simulink model "Scenario_3_PF"  (R2020b)
settings: Solver=ode1  StartTime=0.0  StopTime=10.0  RelTol=1e-3
InitFcn:
  | Scenario_3_parameters;
values from neighbouring files (symbols this model uses):
  c0 = c0_zeb    (= 6.57988e-09)    [Scenario_17_parameters_v2.m]    (also in Scenario_1_parameters_v2.m; Scenario_2_parameters_v2.m; Scenario_3_parameters_v2.m)
  c0_hawk = 6.37282e-09    [Scenario_17_parameters_v2.m]    (also in Scenario_1_parameters_v2.m; Scenario_2_parameters_v2.m; Scenario_3_parameters_v2.m)
  c1 = c1_zeb    (= 9.15905e-09)    [Scenario_17_parameters_v2.m]    (also in Scenario_1_parameters_v2.m; Scenario_2_parameters_v2.m; Scenario_3_parameters_v2.m)
  c1_hawk = 8.76156e-09    [Scenario_17_parameters_v2.m]    (also in Scenario_1_parameters_v2.m; Scenario_2_parameters_v2.m; Scenario_3_parameters_v2.m)
  fg = 50    [Scenario_17_parameters_v2.m]    (also in Scenario_1_parameters_v2.m; Scenario_2_parameters_v2.m; Scenario_3_parameters_v2.m)
  G10gen = 0.90    (= 0.9)    [Scenario_3_parameters_v2.m]
  G12gen = 0.85    [Scenario_3_parameters_v2.m]
  G1gen = 0.4692    [Scenario_17_parameters_v2.m]    (also in Scenario_1_parameters_v2.m = 0.1; Scenario_2_parameters_v2.m = 0.298581; Scenario_3_parameters_v2.m = 0.65)
  G2gen = 0.80    (= 0.8)    [Scenario_1_parameters_v2.m]    (also in Scenario_2_parameters_v2.m = 0.7; Scenario_3_parameters_v2.m = 0.4)
  G3gen = 0.85    [Scenario_1_parameters_v2.m]    (also in Scenario_2_parameters_v2.m = 0.9; Scenario_3_parameters_v2.m = 0.6)
  G4gen = 0.65    [Scenario_3_parameters_v2.m]
  G5gen = 0.75    [Scenario_17_parameters_v2.m]    (also in Scenario_1_parameters_v2.m = 0.8; Scenario_2_parameters_v2.m = 0.8; Scenario_3_parameters_v2.m = 0.705)
  G6gen = 0.90    (= 0.9)    [Scenario_17_parameters_v2.m]    (also in Scenario_1_parameters_v2.m; Scenario_2_parameters_v2.m = 0.81797; Scenario_3_parameters_v2.m = 0.45)
  G7gen = 0.20    (= 0.2)    [Scenario_17_parameters_v2.m]    (also in Scenario_1_parameters_v2.m = 0.5227; Scenario_2_parameters_v2.m = 0.5098; Scenario_3_parameters_v2.m = 0.4)
  G8gen = 0.58    [Scenario_17_parameters_v2.m]    (also in Scenario_3_parameters_v2.m = 0.65)
  G9gen = 0.8833    [Scenario_17_parameters_v2.m]    (also in Scenario_3_parameters_v2.m = 0.9)
  Ihvpk = Ihv*sqrt(2)    [Scenario_17_parameters_v2.m]    (also in Scenario_1_parameters_v2.m; Scenario_2_parameters_v2.m; Scenario_3_parameters_v2.m)
  l0 = l0_zeb    (= 0.00368)    [Scenario_17_parameters_v2.m]    (also in Scenario_1_parameters_v2.m; Scenario_2_parameters_v2.m; Scenario_3_parameters_v2.m)
  l0_hawk = 0.00373    [Scenario_17_parameters_v2.m]    (also in Scenario_1_parameters_v2.m; Scenario_2_parameters_v2.m; Scenario_3_parameters_v2.m)
  l1 = l1_zeb    (= 0.00128)    [Scenario_17_parameters_v2.m]    (also in Scenario_1_parameters_v2.m; Scenario_2_parameters_v2.m; Scenario_3_parameters_v2.m)
  L10dem = 0.04    [Scenario_3_parameters_v2.m]
  L12dem = 0.01    [Scenario_17_parameters_v2.m]    (also in Scenario_3_parameters_v2.m = 0.02)
  L13dem = 0.01    [Scenario_3_parameters_v2.m]
  l1_hawk = 0.00133    [Scenario_17_parameters_v2.m]    (also in Scenario_1_parameters_v2.m; Scenario_2_parameters_v2.m; Scenario_3_parameters_v2.m)
  L1dem = 0.25    [Scenario_17_parameters_v2.m]    (also in Scenario_3_parameters_v2.m = 0.1)
  L3dem = 0.30    (= 0.3)    [Scenario_17_parameters_v2.m]    (also in Scenario_1_parameters_v2.m = 0.1; Scenario_2_parameters_v2.m = 0.1; Scenario_3_parameters_v2.m = 0.2)
  L6dem = 0.15    [Scenario_1_parameters_v2.m]    (also in Scenario_2_parameters_v2.m; Scenario_3_parameters_v2.m = 0.1)
  L7dem = 0.10    (= 0.1)    [Scenario_1_parameters_v2.m]    (also in Scenario_2_parameters_v2.m; Scenario_3_parameters_v2.m = 0.2)
  L9dem = 0.15    [Scenario_17_parameters_v2.m]    (also in Scenario_3_parameters_v2.m = 0.1)
  Pr = Sr*PF    (= 1600500000)    [Scenario_17_parameters_v2.m]    (also in Scenario_1_parameters_v2.m = 1472500000; Scenario_2_parameters_v2.m = 1805000000; Scenario_3_parameters_v2.m = 12740000000)
  Qr = sqrt(Sr^2 - Pr^2)    [Scenario_17_parameters_v2.m]    (also in Scenario_1_parameters_v2.m; Scenario_2_parameters_v2.m; Scenario_3_parameters_v2.m)
  r0 = r0_zeb    (= 0.39362)    [Scenario_17_parameters_v2.m]    (also in Scenario_1_parameters_v2.m; Scenario_2_parameters_v2.m; Scenario_3_parameters_v2.m)
  r0_hawk = 0.44587    [Scenario_17_parameters_v2.m]    (also in Scenario_1_parameters_v2.m; Scenario_2_parameters_v2.m; Scenario_3_parameters_v2.m)
  r1 = r1_zeb    (= 0.06862)    [Scenario_17_parameters_v2.m]    (also in Scenario_1_parameters_v2.m; Scenario_2_parameters_v2.m; Scenario_3_parameters_v2.m)
  r1_hawk = 0.12087    [Scenario_17_parameters_v2.m]    (also in Scenario_1_parameters_v2.m; Scenario_2_parameters_v2.m; Scenario_3_parameters_v2.m)
  Rtpu = Xtpu/40    (= 0.0025)    [Scenario_17_parameters_v2.m]    (also in Scenario_1_parameters_v2.m = 0.00375; Scenario_2_parameters_v2.m = 0.00375; Scenario_3_parameters_v2.m)
  S10non = 500e6    (= 500000000)    [Scenario_3_parameters_v2.m]
  S12non = 250e6    (= 250000000)    [Scenario_3_parameters_v2.m]
  S1non = 700e6    (= 700000000)    [Scenario_17_parameters_v2.m]    (also in Scenario_1_parameters_v2.m = 400000000; Scenario_2_parameters_v2.m = 400000000; Scenario_3_parameters_v2.m = 1000000000)
  S2non = 300e6    (= 300000000)    [Scenario_1_parameters_v2.m]    (also in Scenario_2_parameters_v2.m; Scenario_3_parameters_v2.m = 3000000000)
  S3non = 200e6    (= 200000000)    [Scenario_1_parameters_v2.m]    (also in Scenario_2_parameters_v2.m; Scenario_3_parameters_v2.m = 1000000000)
  S4non = 2000e6    (= 2000000000)    [Scenario_3_parameters_v2.m]
  S5non = 400e6    (= 400000000)    [Scenario_17_parameters_v2.m]    (also in Scenario_1_parameters_v2.m = 500000000; Scenario_2_parameters_v2.m = 500000000; Scenario_3_parameters_v2.m = 2000000000)
  S6non = 150e6    (= 150000000)    [Scenario_17_parameters_v2.m]    (also in Scenario_1_parameters_v2.m = 400000000; Scenario_2_parameters_v2.m = 400000000; Scenario_3_parameters_v2.m = 3000000000)
  S7non = 1500e6    (= 1500000000)    [Scenario_17_parameters_v2.m]    (also in Scenario_1_parameters_v2.m = 200000000; Scenario_2_parameters_v2.m = 200000000; Scenario_3_parameters_v2.m = 4000000000)
  S8non = 600e6    (= 600000000)    [Scenario_17_parameters_v2.m]    (also in Scenario_3_parameters_v2.m = 2000000000)
  S9non = 200e6    (= 200000000)    [Scenario_17_parameters_v2.m]    (also in Scenario_3_parameters_v2.m = 1500000000)
  tonvsc = 0    [Scenario_17_parameters_v2.m]    (also in Scenario_1_parameters_v2.m; Scenario_2_parameters_v2.m; Scenario_3_parameters_v2.m = 0.0001)
  Ts = 50e-6    (= 5e-05)    [Scenario_17_parameters_v2.m]    (also in Scenario_1_parameters_v2.m = 0.0002; Scenario_2_parameters_v2.m = 2e-05; Scenario_3_parameters_v2.m = 0.0001)
  Vhv = 220e3    (= 220000)    [Scenario_17_parameters_v2.m]    (also in Scenario_1_parameters_v2.m; Scenario_2_parameters_v2.m; Scenario_3_parameters_v2.m)
  Vmv = 22e3    (= 22000)    [Scenario_17_parameters_v2.m]    (also in Scenario_1_parameters_v2.m; Scenario_2_parameters_v2.m; Scenario_3_parameters_v2.m)
  wc1 = wsw1/10    (= 848.230016469)    [Scenario_17_parameters_v2.m]    (also in Scenario_1_parameters_v2.m; Scenario_2_parameters_v2.m; Scenario_3_parameters_v2.m)
  wdc1 = wc1/10    (= 84.8230016469)    [Scenario_17_parameters_v2.m]    (also in Scenario_1_parameters_v2.m; Scenario_2_parameters_v2.m; Scenario_3_parameters_v2.m)
  wpq1 = wc1/10    (= 84.8230016469)    [Scenario_17_parameters_v2.m]    (also in Scenario_1_parameters_v2.m; Scenario_2_parameters_v2.m; Scenario_3_parameters_v2.m)
  wsw1 = ksw1*2*pi*fg    (= 8482.30016469)    [Scenario_17_parameters_v2.m]    (also in Scenario_1_parameters_v2.m; Scenario_2_parameters_v2.m; Scenario_3_parameters_v2.m)
  Xtpu = 0.10    (= 0.1)    [Scenario_17_parameters_v2.m]    (also in Scenario_1_parameters_v2.m = 0.15; Scenario_2_parameters_v2.m = 0.15; Scenario_3_parameters_v2.m)
undefined symbols (not defined in the file or in its folder): D11, Delta, Kf, r, theta0
libraries: powerlib x426, simulink_extras x305, powerlib_meascontrol x139, pid_lib x109, eeGeneralControl x72, simulink x60, eeTransforms x54, spsFirstOrderFilterLib x36, eePwmGeneratorTwoLevel x9
(part 1 of 36)
settings Model: Creator=Usuario  LastModifiedBy=Usuario

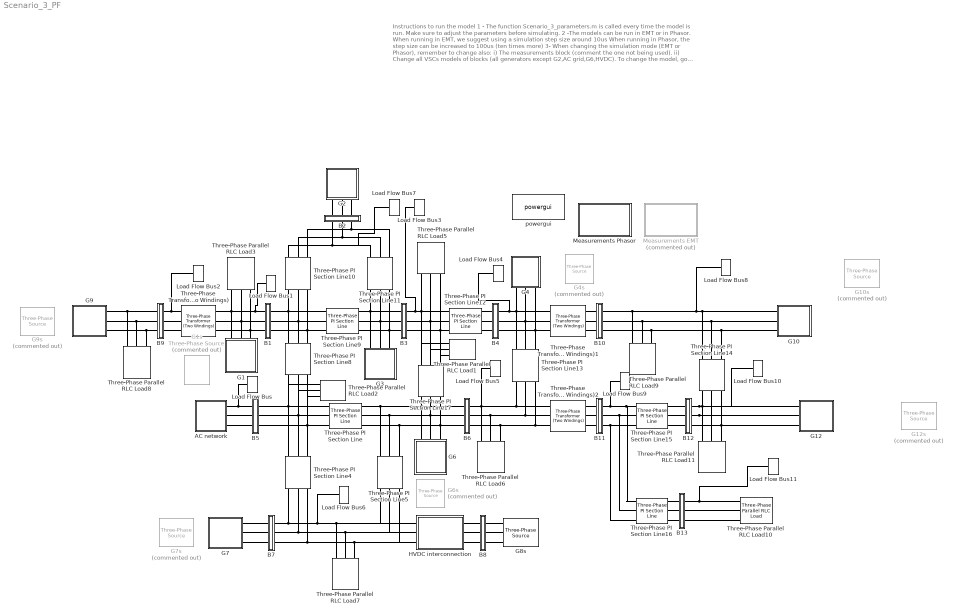
== system Scenario_3_PF ==
  note: Instructions to run the model
      |
      | 1 - The function Scenario_3_parameters.m is called every time the model is run. Make sure to adjust the parameters before simulating.
      | 2 -The models can be run in EMT or in Phasor.
      | 	When running in EMT, we suggest using a simulation step size around 10us
      | 	When running in Phasor, the step size can be increased to 100us (ten times more)
      | 3- When changing the simulation mode (EMT or Phasor), remember to change also:
      | 	i) The measurements block (comment the one not being used).
      | 	ii) Change all VSCs models of blocks (all generators except G2,AC grid,G6,HVDC).
      | 	    To change the model, go to the block VSC and choose one model of droplist under the parameter 'VSC model'
      | 	    We recommend the model AVG model for EMT and the I-ref model for Phasor.
      | 4- The synchronous generators were initialized using power flow to have a near-flat initialization.
      |      As the VSCs are not standard blocks in Simulink, they are not considered in the power flow.
      |     To consider them, connect the voltage source in their place and run the power flow. Then, substitute by the VSCs.
  AC network : Subsystem
      mask Display:
      | disp('SG')
      | %x = [0:0.001:1];
      | %y = 0.2*sin(10*x) + 0.5;
      | %plot(x,y)
  B1 : Subsystem
  B10 : Subsystem
  B11 : Subsystem
  B12 : Subsystem
  B13 : Subsystem
  B2 : Subsystem
  B3 : Subsystem
  B4 : Subsystem
  B5 : Subsystem
  B6 : Subsystem
  B7 : Subsystem
  B8 : Subsystem
  B9 : Subsystem
  G1 : Subsystem
  G10 : Subsystem
  G10s : powerlib/Electrical Sources/Three-Phase Source  Commented=on  InternalConnection=Yg  VoltagePhases=off  Voltage=Vmv  PhaseAngle=-8.2202  Voltage_phases=[25e3 25e3 25e3]/sqrt(3)  PhaseAngles_phases=[0 -120 +120]  Frequency=fg  NonIdealSource=on  SpecifyImpedance=off  Resistance=0.0036  Inductance=4.6219e-04  ShortCircuitLevel=100e6  BaseVoltage=Vmv  XRratio=7  BusType=PV  Pref=S10non*G10gen  Qref=0  Prefabc=[10e3, 10e3, 10e3]  Qrefabc=[0, 0, 0]  Qmin=-inf  Qmax=inf
  G12 : Subsystem
  G12s : powerlib/Electrical Sources/Three-Phase Source  Commented=on  InternalConnection=Yg  VoltagePhases=off  Voltage=Vmv  PhaseAngle=-8.2202  Voltage_phases=[25e3 25e3 25e3]/sqrt(3)  PhaseAngles_phases=[0 -120 +120]  Frequency=fg  NonIdealSource=on  SpecifyImpedance=off  Resistance=0.0012  Inductance=1.5406e-04  ShortCircuitLevel=100e6  BaseVoltage=Vmv  XRratio=7  BusType=PV  Pref=S12non*G12gen  Qref=0  Prefabc=[10e3, 10e3, 10e3]  Qrefabc=[0, 0, 0]  Qmin=-inf  Qmax=inf
  G1s : powerlib/Electrical Sources/Three-Phase Source  Commented=on  InternalConnection=Yg  VoltagePhases=off  Voltage=(220000)*1.15627  PhaseAngle=-32.4209  Voltage_phases=[25e3 25e3 25e3]/sqrt(3)  PhaseAngles_phases=[0 -120 +120]  Frequency=fg  NonIdealSource=on  SpecifyImpedance=off  Resistance=0.1815  Inductance=0.0231  ShortCircuitLevel=100e6  BaseVoltage=Vhv  XRratio=7  BusType=PV  Pref=S1non*G1gen  Qref=0  Prefabc=[10e3, 10e3, 10e3]  Qrefabc=[0, 0, 0]  Qmin=-inf  Qmax=inf
  G2 : Subsystem
      mask Display: disp('SG')
  G3 : Subsystem
      mask Display:
      | disp('SG')
      | %x = [0:0.001:1];
      | %y = 0.2*sin(10*x) + 0.5;
      | %plot(x,y)
  G4 : Subsystem
  G4s : powerlib/Electrical Sources/Three-Phase Source  Commented=on  InternalConnection=Yg  VoltagePhases=off  Voltage=(220000)*1.03369  PhaseAngle=34.3009  Voltage_phases=[25e3 25e3 25e3]/sqrt(3)  PhaseAngles_phases=[0 -120 +120]  Frequency=fg  NonIdealSource=on  SpecifyImpedance=off  Resistance=0.0907  Inductance=0.0116  ShortCircuitLevel=100e6  BaseVoltage=Vhv  XRratio=7  BusType=PV  Pref=S4non*G4gen  Qref=0  Prefabc=[10e3, 10e3, 10e3]  Qrefabc=[0, 0, 0]  Qmin=-inf  Qmax=inf
  G6 : Subsystem
  G6s : powerlib/Electrical Sources/Three-Phase Source  Commented=on  InternalConnection=Yg  VoltagePhases=off  Voltage=(220000)*1.04844  PhaseAngle=25.567  Voltage_phases=[25e3 25e3 25e3]/sqrt(3)  PhaseAngles_phases=[0 -120 +120]  Frequency=fg  NonIdealSource=on  SpecifyImpedance=off  Resistance=0.0605  Inductance=0.0077  ShortCircuitLevel=100e6  BaseVoltage=Vhv  XRratio=7  BusType=PV  Pref=S6non*G6gen  Qref=0  Prefabc=[10e3, 10e3, 10e3]  Qrefabc=[0, 0, 0]  Qmin=-inf  Qmax=inf
  G7 : Subsystem
  G7s : powerlib/Electrical Sources/Three-Phase Source  Commented=on  InternalConnection=Yg  VoltagePhases=off  Voltage=(220000)*1.02099  PhaseAngle=19.4593  Voltage_phases=[25e3 25e3 25e3]/sqrt(3)  PhaseAngles_phases=[0 -120 +120]  Frequency=fg  NonIdealSource=on  SpecifyImpedance=off  Resistance=0.0454  Inductance=0.0058  ShortCircuitLevel=100e6  BaseVoltage=Vhv  XRratio=7  BusType=PV  Pref=S7non*G7gen  Qref=0  Prefabc=[10e3, 10e3, 10e3]  Qrefabc=[0, 0, 0]  Qmin=-inf  Qmax=inf
  G8s : powerlib/Electrical Sources/Three-Phase Source  InternalConnection=Yg  VoltagePhases=off  Voltage=Vhv  PhaseAngle=0  Voltage_phases=[25e3 25e3 25e3]/sqrt(3)  PhaseAngles_phases=[0 -120 +120]  Frequency=fg  NonIdealSource=on  SpecifyImpedance=off  Resistance=0.0907  Inductance=0.0116  ShortCircuitLevel=100e6  BaseVoltage=Vhv  XRratio=7  BusType=PV  Pref=S8non*G8gen  Qref=0  Prefabc=[10e3, 10e3, 10e3]  Qrefabc=[0, 0, 0]  Qmin=-inf  Qmax=inf
  G9 : Subsystem
  G9s : powerlib/Electrical Sources/Three-Phase Source  Commented=on  InternalConnection=Yg  VoltagePhases=off  Voltage=(22000)*1.0541  PhaseAngle=-34.6795  Voltage_phases=[25e3 25e3 25e3]/sqrt(3)  PhaseAngles_phases=[0 -120 +120]  Frequency=fg  NonIdealSource=on  SpecifyImpedance=off  Resistance=0.0012  Inductance=1.5406e-04  ShortCircuitLevel=100e6  BaseVoltage=Vmv  XRratio=7  BusType=PV  Pref=S9non*G9gen  Qref=0  Prefabc=[10e3, 10e3, 10e3]  Qrefabc=[0, 0, 0]  Qmin=-inf  Qmax=inf
  HVDC interconnection : Subsystem
  Load Flow Bus : powerlib/Measurements/Load Flow Bus  LConnTagsString=a  Phases=single  Connectors=on one side  ID=BUS_5  Vbase=Vhv  Vref=1  Vangle=0  VLF=1.006  VLFb=1  VLFc=1  angleLF=-24.79  angleLFb=0  angleLFc=0
  Load Flow Bus1 : powerlib/Measurements/Load Flow Bus  LConnTagsString=a  Phases=single  Connectors=on one side  ID=BUS_1  Vbase=Vhv  Vref=1  Vangle=0  VLF=1  VLFb=1  VLFc=1  angleLF=-35.58  angleLFb=0  angleLFc=0
  Load Flow Bus10 : powerlib/Measurements/Load Flow Bus  LConnTagsString=a  Phases=single  Connectors=on one side  ID=BUS_12  Vbase=Vmv  Vref=1  Vangle=0  VLF=0.06031  VLFb=1  VLFc=1  angleLF=-140.6  angleLFb=0  angleLFc=0
  Load Flow Bus11 : powerlib/Measurements/Load Flow Bus  LConnTagsString=a  Phases=single  Connectors=on one side  ID=BUS_13  Vbase=Vmv  Vref=1  Vangle=0  VLF=0.05913  VLFb=1  VLFc=1  angleLF=-127.7  angleLFb=0  angleLFc=0
  Load Flow Bus2 : powerlib/Measurements/Load Flow Bus  LConnTagsString=a  Phases=single  Connectors=on one side  ID=BUS_9  Vbase=Vmv  Vref=1  Vangle=0  VLF=1  VLFb=1  VLFc=1  angleLF=-39.1  angleLFb=0  angleLFc=0
  Load Flow Bus3 : powerlib/Measurements/Load Flow Bus  LConnTagsString=a  Phases=single  Connectors=on one side  ID=BUS_3  Vbase=Vhv  Vref=1  Vangle=0  VLF=0.9499  VLFb=1  VLFc=1  angleLF=-5.136  angleLFb=0  angleLFc=0
  Load Flow Bus4 : powerlib/Measurements/Load Flow Bus  LConnTagsString=a  Phases=single  Connectors=on one side  ID=BUS_4  Vbase=Vhv  Vref=1  Vangle=0  VLF=1  VLFb=1  VLFc=1  angleLF=26.37  angleLFb=0  angleLFc=0
  Load Flow Bus5 : powerlib/Measurements/Load Flow Bus  LConnTagsString=a  Phases=single  Connectors=on one side  ID=BUS_6  Vbase=Vhv  Vref=1  Vangle=0  VLF=1  VLFb=1  VLFc=1  angleLF=17.81  angleLFb=0  angleLFc=0
  Load Flow Bus6 : powerlib/Measurements/Load Flow Bus  LConnTagsString=a  Phases=single  Connectors=on one side  ID=BUS_7  Vbase=Vhv  Vref=1  Vangle=0  VLF=1  VLFb=1  VLFc=1  angleLF=15.25  angleLFb=0  angleLFc=0
  Load Flow Bus7 : powerlib/Measurements/Load Flow Bus  LConnTagsString=a  Phases=single  Connectors=on one side  ID=BUS_2  Vbase=Vhv  Vref=1  Vangle=0  VLF=0.9954  VLFb=1  VLFc=1  angleLF=-6.449  angleLFb=0  angleLFc=0
  Load Flow Bus8 : powerlib/Measurements/Load Flow Bus  LConnTagsString=a  Phases=single  Connectors=on one side  ID=BUS_10  Vbase=Vmv  Vref=1  Vangle=0  VLF=0.4409  VLFb=1  VLFc=1  angleLF=-103.7  angleLFb=0  angleLFc=0
  Load Flow Bus9 : powerlib/Measurements/Load Flow Bus  LConnTagsString=a  Phases=single  Connectors=on one side  ID=BUS_11  Vbase=Vmv  Vref=1  Vangle=0  VLF=0.4051  VLFb=1  VLFc=1  angleLF=-78.99  angleLFb=0  angleLFc=0
  Measurements EMT : Subsystem  Commented=on
  Measurements Phasor : Subsystem
  Three-Phase PI Section Line : powerlib/Elements/Three-Phase PI Section Line  LConnTagsString=a|b|c  RConnTagsString=A|B|C  Length=80  Frequency=fg  Resistances=[r1 r0]  Inductances="[l1  l0]"  Capacitances=[c1 c0]
  Three-Phase PI Section Line10 : powerlib/Elements/Three-Phase PI Section Line  LConnTagsString=a|b|c  RConnTagsString=A|B|C  Length=100  Frequency=fg  Resistances=[r1 r0]  Inductances="[l1  l0]"  Capacitances=[c1 c0]
  Three-Phase PI Section Line11 : powerlib/Elements/Three-Phase PI Section Line  LConnTagsString=a|b|c  RConnTagsString=A|B|C  Length=70  Frequency=fg  Resistances=[r1 r0]  Inductances="[l1  l0]"  Capacitances=[c1 c0]
  Three-Phase PI Section Line12 : powerlib/Elements/Three-Phase PI Section Line  LConnTagsString=a|b|c  RConnTagsString=A|B|C  Length=40  Frequency=fg  Resistances=[r1 r0]  Inductances="[l1  l0]"  Capacitances=[c1 c0]
  Three-Phase PI Section Line{4,8,13,17} (4 alike) : powerlib/Elements/Three-Phase PI Section Line  LConnTagsString=a|b|c  RConnTagsString=A|B|C  Length=50  Frequency=fg  Resistances=[r1 r0]  Inductances="[l1  l0]"  Capacitances=[c1 c0]
  Three-Phase PI Section Line14 : powerlib/Elements/Three-Phase PI Section Line  LConnTagsString=a|b|c  RConnTagsString=A|B|C  Length=20  Frequency=fg  Resistances=[r1_hawk r0_hawk]  Inductances="[l1_hawk  l0_hawk]"  Capacitances=[c1_hawk c0_hawk]
  Three-Phase PI Section Line15 : powerlib/Elements/Three-Phase PI Section Line  LConnTagsString=a|b|c  RConnTagsString=A|B|C  Length=20  Frequency=fg  Resistances=[r1_hawk r0_hawk]  Inductances="[l1_hawk  l0_hawk]"  Capacitances=[c1_hawk c0_hawk]
  Three-Phase PI Section Line16 : powerlib/Elements/Three-Phase PI Section Line  LConnTagsString=a|b|c  RConnTagsString=A|B|C  Length=10  Frequency=fg  Resistances=[r1_hawk r0_hawk]  Inductances="[l1_hawk  l0_hawk]"  Capacitances=[c1_hawk c0_hawk]
  Three-Phase PI Section Line5 : powerlib/Elements/Three-Phase PI Section Line  LConnTagsString=a|b|c  RConnTagsString=A|B|C  Length=100  Frequency=fg  Resistances=[r1 r0]  Inductances="[l1  l0]"  Capacitances=[c1 c0]
  Three-Phase PI Section Line9 : powerlib/Elements/Three-Phase PI Section Line  LConnTagsString=a|b|c  RConnTagsString=A|B|C  Length=80  Frequency=fg  Resistances=[r1 r0]  Inductances="[l1  l0]"  Capacitances=[c1 c0]
  Three-Phase Parallel RLC Load1 : powerlib/Elements/Three-Phase Parallel RLC Load  LConnTagsString=A|B|C  Configuration=Y (grounded)  NominalVoltage=Vhv  Vabc=[1e3 1e3 1e3]  Vabcp=[1e3 1e3 1e3]  NominalFrequency=fg  UnbalancedPower=off  ActivePower=0  InductivePower=0  CapacitivePower=800e6  Pabc=[10e3 9e3 11e3]  QLabc=[100 90 110]  QCabc=[100 90 110]  Pabcp=[10e3 9e3 11e3]  QLabcp=[100 90 110]  QCabcp=[100 90 110]  Measurements=None  LoadType=constant Z
  Three-Phase Parallel RLC Load10 : powerlib/Elements/Three-Phase Parallel RLC Load  LConnTagsString=A|B|C  Configuration=Y (grounded)  NominalVoltage=Vmv  Vabc=[1e3 1e3 1e3]  Vabcp=[1e3 1e3 1e3]  NominalFrequency=fg  UnbalancedPower=off  ActivePower=Pr*L13dem  InductivePower=0  CapacitivePower=0  Pabc=[10e3 9e3 11e3]  QLabc=[100 90 110]  QCabc=[100 90 110]  Pabcp=[10e3 9e3 11e3]  QLabcp=[100 90 110]  QCabcp=[100 90 110]  Measurements=None  LoadType=constant Z
  Three-Phase Parallel RLC Load11 : powerlib/Elements/Three-Phase Parallel RLC Load  LConnTagsString=A|B|C  Configuration=Y (grounded)  NominalVoltage=Vmv  Vabc=[1e3 1e3 1e3]  Vabcp=[1e3 1e3 1e3]  NominalFrequency=fg  UnbalancedPower=off  ActivePower=Pr*L12dem  InductivePower=Qr*L12dem  CapacitivePower=0  Pabc=[10e3 9e3 11e3]  QLabc=[100 90 110]  QCabc=[100 90 110]  Pabcp=[10e3 9e3 11e3]  QLabcp=[100 90 110]  QCabcp=[100 90 110]  Measurements=None  LoadType=constant Z
  Three-Phase Parallel RLC Load2 : powerlib/Elements/Three-Phase Parallel RLC Load  LConnTagsString=A|B|C  Configuration=Y (grounded)  NominalVoltage=Vhv  Vabc=[1e3 1e3 1e3]  Vabcp=[1e3 1e3 1e3]  NominalFrequency=fg  UnbalancedPower=off  ActivePower=0  InductivePower=0  CapacitivePower=500e6  Pabc=[10e3 9e3 11e3]  QLabc=[100 90 110]  QCabc=[100 90 110]  Pabcp=[10e3 9e3 11e3]  QLabcp=[100 90 110]  QCabcp=[100 90 110]  Measurements=None  LoadType=constant Z
  Three-Phase Parallel RLC Load3 : powerlib/Elements/Three-Phase Parallel RLC Load  LConnTagsString=A|B|C  Configuration=Y (grounded)  NominalVoltage=Vhv  Vabc=[1e3 1e3 1e3]  Vabcp=[1e3 1e3 1e3]  NominalFrequency=fg  UnbalancedPower=off  ActivePower=Pr*L1dem  InductivePower=Qr*L1dem  CapacitivePower=0  Pabc=[10e3 9e3 11e3]  QLabc=[100 90 110]  QCabc=[100 90 110]  Pabcp=[10e3 9e3 11e3]  QLabcp=[100 90 110]  QCabcp=[100 90 110]  Measurements=None  LoadType=constant Z
  Three-Phase Parallel RLC Load5 : powerlib/Elements/Three-Phase Parallel RLC Load  LConnTagsString=A|B|C  Configuration=Y (grounded)  NominalVoltage=Vhv  Vabc=[1e3 1e3 1e3]  Vabcp=[1e3 1e3 1e3]  NominalFrequency=fg  UnbalancedPower=off  ActivePower=Pr*L3dem  InductivePower=Qr*L3dem  CapacitivePower=0  Pabc=[10e3 9e3 11e3]  QLabc=[100 90 110]  QCabc=[100 90 110]  Pabcp=[10e3 9e3 11e3]  QLabcp=[100 90 110]  QCabcp=[100 90 110]  Measurements=None  LoadType=constant Z
  Three-Phase Parallel RLC Load6 : powerlib/Elements/Three-Phase Parallel RLC Load  LConnTagsString=A|B|C  Configuration=Y (grounded)  NominalVoltage=Vhv  Vabc=[1e3 1e3 1e3]  Vabcp=[1e3 1e3 1e3]  NominalFrequency=fg  UnbalancedPower=off  ActivePower=Pr*L6dem  InductivePower=Qr*L6dem  CapacitivePower=0  Pabc=[10e3 9e3 11e3]  QLabc=[100 90 110]  QCabc=[100 90 110]  Pabcp=[10e3 9e3 11e3]  QLabcp=[100 90 110]  QCabcp=[100 90 110]  Measurements=None  LoadType=constant Z
  Three-Phase Parallel RLC Load7 : powerlib/Elements/Three-Phase Parallel RLC Load  LConnTagsString=A|B|C  Configuration=Y (grounded)  NominalVoltage=Vhv  Vabc=[1e3 1e3 1e3]  Vabcp=[1e3 1e3 1e3]  NominalFrequency=fg  UnbalancedPower=off  ActivePower=Pr*L7dem  InductivePower=Qr*L7dem  CapacitivePower=0  Pabc=[10e3 9e3 11e3]  QLabc=[100 90 110]  QCabc=[100 90 110]  Pabcp=[10e3 9e3 11e3]  QLabcp=[100 90 110]  QCabcp=[100 90 110]  Measurements=None  LoadType=constant Z
  Three-Phase Parallel RLC Load8 : powerlib/Elements/Three-Phase Parallel RLC Load  LConnTagsString=A|B|C  Configuration=Y (grounded)  NominalVoltage=Vmv  Vabc=[1e3 1e3 1e3]  Vabcp=[1e3 1e3 1e3]  NominalFrequency=fg  UnbalancedPower=off  ActivePower=Pr*L9dem  InductivePower=Qr*L9dem  CapacitivePower=0  Pabc=[10e3 9e3 11e3]  QLabc=[100 90 110]  QCabc=[100 90 110]  Pabcp=[10e3 9e3 11e3]  QLabcp=[100 90 110]  QCabcp=[100 90 110]  Measurements=None  LoadType=constant Z
  Three-Phase Parallel RLC Load9 : powerlib/Elements/Three-Phase Parallel RLC Load  LConnTagsString=A|B|C  Configuration=Y (grounded)  NominalVoltage=Vmv  Vabc=[1e3 1e3 1e3]  Vabcp=[1e3 1e3 1e3]  NominalFrequency=fg  UnbalancedPower=off  ActivePower=Pr*L10dem  InductivePower=Qr*L10dem  CapacitivePower=0  Pabc=[10e3 9e3 11e3]  QLabc=[100 90 110]  QCabc=[100 90 110]  Pabcp=[10e3 9e3 11e3]  QLabcp=[100 90 110]  QCabcp=[100 90 110]  Measurements=None  LoadType=constant Z
  Three-Phase Transformer (Two Windings) : powerlib/Elements/Three-Phase Transformer (Two Windings)  Winding1Connection=Yg  Winding2Connection=Yg  CoreType=Three single-phase transformers  SetSaturation=off  Hysteresis=off  DataFile='hysteresis'  SetInitialFlux=off  Measurements=None  UNITS=pu  NominalPower=[S9non , fg ]  Winding1=[Vmv 0.00125 0.05]  Winding2=[Vhv 0.00125 0.05]  Rm=5000  Lm=5000  L0=0.5  Saturation=[ 0,0 ; 0.0024,1.2 ; 1.0,1.52 ]  InitialFluxes=[ 0.8 , -0.8 , 0.7 ]  BreakLoop=off  DiscreteSolver=Trapezoidal iterative  DataType=off  TransfoNumber=1
  Three-Phase Transformer (Two Windings)1 : powerlib/Elements/Three-Phase Transformer (Two Windings)  Winding1Connection=Yg  Winding2Connection=Yg  CoreType=Three single-phase transformers  SetSaturation=off  Hysteresis=off  DataFile='hysteresis'  SetInitialFlux=off  Measurements=None  UNITS=pu  NominalPower=[S10non , fg ]  Winding1=[Vhv 0.00125 0.05]  Winding2=[Vmv 0.00125 0.05]  Rm=5000  Lm=5000  L0=0.5  Saturation=[ 0,0 ; 0.0024,1.2 ; 1.0,1.52 ]  InitialFluxes=[ 0.8 , -0.8 , 0.7 ]  BreakLoop=off  DiscreteSolver=Trapezoidal iterative  DataType=off  TransfoNumber=1
  Three-Phase Transformer (Two Windings)2 : powerlib/Elements/Three-Phase Transformer (Two Windings)  Winding1Connection=Yg  Winding2Connection=Yg  CoreType=Three single-phase transformers  SetSaturation=off  Hysteresis=off  DataFile='hysteresis'  SetInitialFlux=off  Measurements=None  UNITS=pu  NominalPower=[S12non , fg ]  Winding1=[Vhv 0.00125 0.05]  Winding2=[Vmv 0.00125 0.05]  Rm=5000  Lm=5000  L0=0.5  Saturation=[ 0,0 ; 0.0024,1.2 ; 1.0,1.52 ]  InitialFluxes=[ 0.8 , -0.8 , 0.7 ]  BreakLoop=off  DiscreteSolver=Trapezoidal iterative  DataType=off  TransfoNumber=1
  powergui : powerlib/powergui  Priority=1  SimulationMode=Discrete phasor  SampleTime=Ts  frequency=fg  Iterations=50  frequencyindice=50  Pbase=100e6  ErrMax=0.0001  UnitsV=kV  UnitsW=MW  buscounter=0  FunctionMessages=off  echomessages=off  EnableUseOfTLC=off  CurrentSourceSwitches=off  DisableSnubberDevices=off  DisableRonSwitches=off  DisableVfSwitches=off  DisplayEquations=off  AutomaticDiscreteSolvers=off  SolverType=Tustin/Backward Euler (TBE)  Interpol=off  ExternalGateDelay=off  methode=off  Ts=100  x0status=blocks  SPID=on  SwTol=0  HookPort=off  NonlinearTolerance=1e-4  nMaxIteration=100  ContinueOnMaxIteration=off  RestoreLinks=warning  ResistiveCurrentMeasurement=off  Frange=[0:2:500]  Ylog=off  Xlog=on  ShowGrid=off  save=off  variable=ZData  structure=0  ZoomFFT=off  StartTime=0.0  cycles=1  DisplayStyle=1  fundamental=60  FreqAxis=off  MaxFrequency=1000  frequencyindicesteady=1  RmsSteady=2  display=off
  connections:
  AC network/RConn1 -- B5/LConn1 -- Load Flow Bus/LConn1
  AC network/RConn2 -- B5/LConn2
  AC network/RConn3 -- B5/LConn3
  Three-Phase PI Section Line/LConn1 -- Three-Phase Parallel RLC Load2/LConn1 -- Three-Phase PI Section Line8/LConn1 -- Three-Phase PI Section Line4/RConn1 -- B5/RConn1
  Three-Phase PI Section Line/LConn2 -- Three-Phase Parallel RLC Load2/LConn2 -- Three-Phase PI Section Line8/LConn2 -- B5/RConn2 -- Three-Phase PI Section Line4/RConn2
  Three-Phase PI Section Line/LConn3 -- Three-Phase PI Section Line8/LConn3 -- Three-Phase Parallel RLC Load2/LConn3 -- Three-Phase PI Section Line4/RConn3 -- B5/RConn3
  B6/LConn1 -- Three-Phase PI Section Line/RConn1 -- Three-Phase PI Section Line5/RConn1 -- G6/RConn1 -- Three-Phase PI Section Line17/RConn1
  B6/LConn2 -- Three-Phase PI Section Line/RConn2 -- Three-Phase PI Section Line5/RConn2 -- G6/RConn2 -- Three-Phase PI Section Line17/RConn2
  B7/RConn1 -- Load Flow Bus6/LConn1 -- Three-Phase PI Section Line5/LConn1 -- HVDC interconnection/LConn1 -- Three-Phase Parallel RLC Load7/LConn1 -- Three-Phase PI Section Line4/LConn1
  Three-Phase PI Section Line4/LConn2 -- Three-Phase PI Section Line5/LConn2 -- HVDC interconnection/LConn2 -- Three-Phase Parallel RLC Load7/LConn2 -- B7/RConn2
  Three-Phase PI Section Line4/LConn3 -- Three-Phase PI Section Line5/LConn3 -- HVDC interconnection/LConn3 -- Three-Phase Parallel RLC Load7/LConn3 -- B7/RConn3
  Three-Phase PI Section Line9/LConn1 -- Three-Phase PI Section Line10/LConn1 -- Three-Phase PI Section Line8/RConn1 -- B1/RConn1
  Three-Phase PI Section Line9/LConn2 -- Three-Phase PI Section Line10/LConn2 -- Three-Phase PI Section Line8/RConn2 -- B1/RConn2
  Three-Phase PI Section Line9/LConn3 -- Three-Phase PI Section Line10/LConn3 -- Three-Phase PI Section Line8/RConn3 -- B1/RConn3
  Three-Phase Transformer (Two Windings)/RConn1 -- G1/RConn1 -- Load Flow Bus1/LConn1 -- B1/LConn1 -- Three-Phase Parallel RLC Load3/LConn1
  Three-Phase Transformer (Two Windings)/RConn2 -- G1/RConn2 -- B1/LConn2 -- Three-Phase Parallel RLC Load3/LConn2
  Three-Phase Transformer (Two Windings)/RConn3 -- Three-Phase Parallel RLC Load3/LConn3 -- G1/RConn3 -- B1/LConn3
  B9/RConn1 -- Load Flow Bus2/LConn1 -- Three-Phase Transformer (Two Windings)/LConn1
  B9/RConn2 -- Three-Phase Transformer (Two Windings)/LConn2
  B9/RConn3 -- Three-Phase Transformer (Two Windings)/LConn3
  Three-Phase Parallel RLC Load8/LConn1 -- G9/RConn1 -- B9/LConn1
  Three-Phase Parallel RLC Load8/LConn2 -- G9/RConn2 -- B9/LConn2
  Three-Phase Parallel RLC Load8/LConn3 -- G9/RConn3 -- B9/LConn3
  B2/RConn1 -- Load Flow Bus7/LConn1 -- Three-Phase PI Section Line11/RConn1 -- Three-Phase PI Section Line10/RConn1
  B2/RConn2 -- Three-Phase PI Section Line10/RConn2 -- Three-Phase PI Section Line11/RConn2
  B2/RConn3 -- Three-Phase PI Section Line10/RConn3 -- Three-Phase PI Section Line11/RConn3
  G2/RConn1 -- B2/LConn1
  G2/RConn2 -- B2/LConn2
  G2/RConn3 -- B2/LConn3
  B3/LConn1 -- G3/RConn1 -- Three-Phase PI Section Line9/RConn1 -- Three-Phase PI Section Line11/LConn1
  B3/LConn2 -- Three-Phase PI Section Line9/RConn2 -- G3/RConn2 -- Three-Phase PI Section Line11/LConn2
  B3/LConn3 -- Three-Phase PI Section Line9/RConn3 -- G3/RConn3 -- Three-Phase PI Section Line11/LConn3
  Three-Phase PI Section Line12/LConn1 -- Three-Phase Parallel RLC Load1/LConn1 -- Three-Phase PI Section Line17/LConn1 -- Three-Phase Parallel RLC Load5/LConn1 -- Load Flow Bus3/LConn1 -- B3/RConn1
  Three-Phase PI Section Line12/LConn2 -- Three-Phase Parallel RLC Load1/LConn2 -- Three-Phase PI Section Line17/LConn2 -- B3/RConn2 -- Three-Phase Parallel RLC Load5/LConn2
  Three-Phase PI Section Line12/LConn3 -- Three-Phase Parallel RLC Load5/LConn3 -- Three-Phase Parallel RLC Load1/LConn3 -- Three-Phase PI Section Line17/LConn3 -- B3/RConn3
  B4/LConn1 -- Three-Phase PI Section Line12/RConn1
  B4/LConn2 -- Three-Phase PI Section Line12/RConn2
  B4/LConn3 -- Three-Phase PI Section Line12/RConn3
  Three-Phase Transformer (Two Windings)1/LConn1 -- Load Flow Bus4/LConn1 -- B4/RConn1 -- G4/RConn1 -- Three-Phase PI Section Line13/LConn1
  Three-Phase Transformer (Two Windings)1/LConn2 -- B4/RConn2 -- G4/RConn2 -- Three-Phase PI Section Line13/LConn2
  Three-Phase Transformer (Two Windings)1/LConn3 -- G4/RConn3 -- B4/RConn3 -- Three-Phase PI Section Line13/LConn3
  B10/LConn1 -- Three-Phase Transformer (Two Windings)1/RConn1
  B10/LConn2 -- Three-Phase Transformer (Two Windings)1/RConn2
  B10/LConn3 -- Three-Phase Transformer (Two Windings)1/RConn3
  Three-Phase Transformer (Two Windings)2/LConn1 -- Load Flow Bus5/LConn1 -- Three-Phase Parallel RLC Load6/LConn1 -- B6/RConn1 -- Three-Phase PI Section Line13/RConn1
  Three-Phase Transformer (Two Windings)2/LConn2 -- Three-Phase PI Section Line13/RConn2 -- Three-Phase Parallel RLC Load6/LConn2 -- B6/RConn2
  Three-Phase Transformer (Two Windings)2/LConn3 -- Three-Phase PI Section Line13/RConn3 -- Three-Phase Parallel RLC Load6/LConn3 -- B6/RConn3
  Three-Phase PI Section Line14/LConn1 -- G10/RConn1 -- B10/RConn1 -- Three-Phase Parallel RLC Load9/LConn1 -- Load Flow Bus8/LConn1
  Three-Phase PI Section Line14/LConn2 -- G10/RConn2 -- B10/RConn2 -- Three-Phase Parallel RLC Load9/LConn2
  Three-Phase PI Section Line14/LConn3 -- G10/RConn3 -- B10/RConn3 -- Three-Phase Parallel RLC Load9/LConn3
  B12/RConn1 -- G12/RConn1 -- Load Flow Bus10/LConn1 -- Three-Phase Parallel RLC Load11/LConn1 -- Three-Phase PI Section Line14/RConn1
  Three-Phase PI Section Line14/RConn3 -- B12/RConn3 -- G12/RConn3 -- Three-Phase Parallel RLC Load11/LConn3
  Three-Phase PI Section Line15/RConn1 -- B12/LConn1
  Three-Phase PI Section Line15/RConn2 -- B12/LConn2
  Three-Phase PI Section Line15/RConn3 -- B12/LConn3
  B11/RConn1 -- Load Flow Bus9/LConn1 -- Three-Phase PI Section Line16/LConn1 -- Three-Phase PI Section Line15/LConn1
  B11/RConn2 -- Three-Phase PI Section Line16/LConn2 -- Three-Phase PI Section Line15/LConn2
  B11/RConn3 -- Three-Phase PI Section Line16/LConn3 -- Three-Phase PI Section Line15/LConn3
  B11/LConn1 -- Three-Phase Transformer (Two Windings)2/RConn1
  B11/LConn2 -- Three-Phase Transformer (Two Windings)2/RConn2
  B11/LConn3 -- Three-Phase Transformer (Two Windings)2/RConn3
  B13/LConn1 -- Three-Phase PI Section Line16/RConn1
  B13/LConn2 -- Three-Phase PI Section Line16/RConn2
  B13/LConn3 -- Three-Phase PI Section Line16/RConn3
  Three-Phase Parallel RLC Load10/LConn1 -- B13/RConn1 -- Load Flow Bus11/LConn1
  Three-Phase Parallel RLC Load10/LConn2 -- B13/RConn2
  Three-Phase Parallel RLC Load10/LConn3 -- B13/RConn3
  B8/RConn1 -- HVDC interconnection/RConn1
  B8/RConn2 -- HVDC interconnection/RConn2
  G8s/RConn1 -- B8/LConn1
  G8s/RConn2 -- B8/LConn2
  G8s/RConn3 -- B8/LConn3
  B8/RConn3 -- HVDC interconnection/RConn3
  B6/LConn3 -- Three-Phase PI Section Line/RConn3 -- Three-Phase PI Section Line5/RConn3 -- G6/RConn3 -- Three-Phase PI Section Line17/RConn3
  B12/RConn2 -- Three-Phase PI Section Line14/RConn2 -- G12/RConn2 -- Three-Phase Parallel RLC Load11/LConn2
  G7/RConn1 -- B7/LConn1
  G7/RConn2 -- B7/LConn2
  G7/RConn3 -- B7/LConn3

== system Scenario_3_PF/AC network ==
  note: Synchronous Machine Model according to ENTSO-E
  note: Nomenclature (according to IEEE Std 421.1-2007):
      | Efd = Exciter output voltage (generator field voltage)
      | Ifd = Exciter output current (generator field current)
      | Vf = Excitation system stabilizer signal
      | Vfe = Signal proportional to exciter field current
      | Vl = Limiters and protective elements feedback
      | Vr = Regulator output
      | Vs = Power System Stabilizer (PSS) output
      | Vsi = Power System Stabilizer (PSS) inputs (shaft speed, frequency, generator electric power, and others
      | Vt = Generator terminal voltage
      | It = Generator terminal current
      | Vref = Voltage regulator reference signal
      | Vc = terminal voltage transducer output
  Bus Selector : BusSelector  OutputSignals=dw,w,vq,vd,iq,id,Peo,Te
  Constant : Constant  Value=G5gen
  Exciter System : Subsystem
  Load Flow Bus : powerlib/Measurements/Load Flow Bus  LConnTagsString=a  Phases=single  Connectors=on one side  ID=BUS_swing  Vbase=Vmv  Vref=1.05  Vangle=0  VLF=1.05  VLFb=1  VLFc=1  angleLF=0  angleLFb=0  angleLFc=0
  Real-Imag to Complex : RealImagToComplex
  Real-Imag to Complex1 : RealImagToComplex
  Ref voltage (p.u) : Constant  Value=1.0
  Snubber : powerlib/Elements/Three-Phase Parallel RLC Load  LConnTagsString=A|B|C  Configuration=Y (grounded)  NominalVoltage=Vmv  Vabc=[1e3 1e3 1e3]  Vabcp=[1e3 1e3 1e3]  NominalFrequency=fg  UnbalancedPower=off  ActivePower=S5non*0.01  InductivePower=0  CapacitivePower=0  Pabc=[10e3 9e3 11e3]  QLabc=[100 90 110]  QCabc=[100 90 110]  Pabcp=[10e3 9e3 11e3]  QLabcp=[100 90 110]  QCabcp=[100 90 110]  Measurements=None  LoadType=constant Z
  Speed Governor : Subsystem  mask{R=0.05, T1=0.5, T2=3, T3=10, Dt=0, Vmin=0, Vmax=10, P0=G5gen}
      mask prompts: R "Controller droop (R)"; T1 "Governor time constant (T1)(sec)"; T2 "Turbine derivative time constant (T2)(sec)"; T3 "Turbine delay time constant (T3)(sec)"; Dt "Frictional losses factor (Dt)"; Vmin "Minimum gate limit (Vmin)(p.u)"; Vmax "Maximum gate limit (Vmax)(p.u)"; P0 "Initial power (p.u)"
      mask Display:
      | disp('TGOV')
      | 
      | port_label('input',1,'Pref')
      | port_label('input',2,'dw')
      | 
      | port_label('output',1,'Pm')
  Synchronous Machine pu Standard : powerlib/Machines/Synchronous Machine pu Standard  PresetModel=No  MechanicalLoad=Mechanical power Pm  ShowDetailedParameters=on  RotorType=Salient-pole  Units=per unit standard parameters  MeasurementBus=on  NominalParameters=[S5non Vmv fg]  Reactances1=[ 1.81, 0.3, 0.23, 1.76, 0.65, 0.25, 0.15 ]  Reactances2=[1.25 0.333 0.292 1.0 0.292 0.15]  dAxisTimeConstants=Open-circuit  qAxisTimeConstants=Open-circuit  TimeConstants1="[5  0.002  0.002]"  TimeConstants2=[ 8.0, 0.03, 1.0, 0.07 ]  TimeConstants3="[  4.49  0.0681  0.0513  ]"  TimeConstants4=[ 8.0, 0.03, 0.3371, 0.0295 ]  TimeConstants5=[ 1.01, 0.053, 0.1 ]  TimeConstants6=[ 1.3201, 0.023, 1.0, 0.07 ]  TimeConstants7=[0.012 0.003 0.003]  TimeConstants8=[ 1.3201, 0.0231, 0.3371, 0.0295 ]  StatorResistance=0.01  Mechanical=[6 0 2]  PolePairs=20  InitialConditions=[0 -120.025 1.02434 1.02434 1.02434 -150.308 -270.308 -30.308 1.5]  SetSaturation=off  Saturation=[0.6404,0.7127,0.8441,0.9214,0.9956,1.082,1.19,1.316,1.457;0.7,0.7698,0.8872,0.9466,0.9969,1.046,1.1,1.151,1.201]  LoadFlowParameters=[2 200000000 0 0 0]  TsPowergui=0  TsBlock=-1  IterativeModel=Trapezoidal non iterative  IterativeDiscreteModel=Trapezoidal non iterative  BusType=swing  Pref=0  Qref=0  Qmin=-inf  Qmax=inf  PLF=0  QLF=0
  Three-Phase Transformer (Two Windings) : powerlib/Elements/Three-Phase Transformer (Two Windings)  Winding1Connection=Delta (D11)  Winding2Connection=Yg  CoreType=Three single-phase transformers  SetSaturation=off  Hysteresis=off  DataFile='hysteresis'  SetInitialFlux=off  Measurements=None  UNITS=pu  NominalPower=[S5non , fg ]  Winding1=[Vmv 0.00125 0.05]  Winding2=[Vhv 0.00125 0.05]  Rm=5000  Lm=5000  L0=0.5  Saturation=[ 0,0 ; 0.0024,1.2 ; 1.0,1.52 ]  InitialFluxes=[ 0.8 , -0.8 , 0.7 ]  BreakLoop=off  DiscreteSolver=Trapezoidal iterative  DataType=off  TransfoNumber=1
  A : PMIOPort  Side=Right
  B : PMIOPort  Port=2  Side=Right
  C : PMIOPort  Port=3  Side=Right
  tag scope: Pe1=global, Te5=global, wm5=global
  wires:
  Bus Selector/1 -> Speed Governor/2(dw), Exciter System/1(<dw>)  "<dw>"
  Bus Selector/4 -> Real-Imag to Complex/2  "<vd>"
  Bus Selector/3 -> Real-Imag to Complex/1  "<vq>"
  Bus Selector/5 -> Real-Imag to Complex1/1  "<iq>"
  Bus Selector/6 -> Real-Imag to Complex1/2  "<id>"
  Real-Imag to Complex/1 -> Exciter System/3(Vt)
  Real-Imag to Complex1/1 -> Exciter System/4(It)
  Bus Selector/8 -> [Te5]  "<Te>"
  Speed Governor/1(Pm) -> Synchronous Machine pu Standard/1
  Exciter System/1(Efd) -> Synchronous Machine pu Standard/2
  Synchronous Machine pu Standard/1 -> Bus Selector/1
  Constant/1 -> Speed Governor/1(RefL)
  Bus Selector/2 -> [wm5]  "<w>"
  Bus Selector/7 -> [Pe1], Exciter System/5(<Peo>)  "<Peo>"
  Ref voltage (p.u)/1 -> Exciter System/2(Vref)
  connections:
  Synchronous Machine pu Standard/RConn1 -- Load Flow Bus/LConn1 -- Three-Phase Transformer (Two Windings)/LConn1 -- Snubber/LConn1
  Synchronous Machine pu Standard/RConn3 -- Three-Phase Transformer (Two Windings)/LConn3 -- Snubber/LConn3
  Synchronous Machine pu Standard/RConn2 -- Three-Phase Transformer (Two Windings)/LConn2 -- Snubber/LConn2
  Three-Phase Transformer (Two Windings)/RConn1 -- A/RConn1
  Three-Phase Transformer (Two Windings)/RConn2 -- B/RConn1
  Three-Phase Transformer (Two Windings)/RConn3 -- C/RConn1

== system Scenario_3_PF/B1 ==
  Current Measurement : powerlib/Measurements/Current Measurement  PhasorSimulation=on  OutputType=Complex  PSBequivalent=0
  Current Measurement1 : powerlib/Measurements/Current Measurement  PhasorSimulation=on  OutputType=Complex  PSBequivalent=0
  Current Measurement2 : powerlib/Measurements/Current Measurement  PhasorSimulation=on  OutputType=Complex  PSBequivalent=0
  Gain : Gain
  Gain1 : Gain
  Ground : powerlib/Elements/Ground  LConnTagsString=a
  Ground1 : powerlib/Elements/Ground  LConnTagsString=a
  Ground2 : powerlib/Elements/Ground  LConnTagsString=a
  Mux : Mux  Inputs=3
  Mux1 : Mux  Inputs=3
  Voltage Measurement : powerlib/Measurements/Voltage Measurement  PhasorSimulation=on  OutputType=Complex  PSBequivalent=0
  Voltage Measurement1 : powerlib/Measurements/Voltage Measurement  PhasorSimulation=on  OutputType=Complex  PSBequivalent=0
  Voltage Measurement2 : powerlib/Measurements/Voltage Measurement  PhasorSimulation=on  OutputType=Complex  PSBequivalent=0
  A : PMIOPort  Side=Left
  B : PMIOPort  Port=2  Side=Left
  C : PMIOPort  Port=3  Side=Left
  a : PMIOPort  Port=4  Side=Right
  b : PMIOPort  Port=5  Side=Right
  c : PMIOPort  Port=6  Side=Right
  tag scope: I1=global, V1=global
  wires:
  Voltage Measurement2/1 -> Mux/3
  Voltage Measurement1/1 -> Mux/2
  Voltage Measurement/1 -> Mux/1
  Current Measurement/1 -> Mux1/1
  Current Measurement1/1 -> Mux1/2
  Current Measurement2/1 -> Mux1/3
  Mux/1 -> Gain/1
  Gain/1 -> [V1]
  Mux1/1 -> Gain1/1
  Gain1/1 -> [I1]
  connections:
  Current Measurement/RConn1 -- a/RConn1
  Current Measurement1/LConn1 -- Voltage Measurement1/LConn1 -- B/RConn1
  Current Measurement2/LConn1 -- Voltage Measurement2/LConn1 -- C/RConn1
  A/RConn1 -- Current Measurement/LConn1 -- Voltage Measurement/LConn1
  Current Measurement1/RConn1 -- b/RConn1
  Current Measurement2/RConn1 -- c/RConn1
  Ground/LConn1 -- Voltage Measurement/LConn2
  Ground1/LConn1 -- Voltage Measurement1/LConn2
  Ground2/LConn1 -- Voltage Measurement2/LConn2

== system Scenario_3_PF/B10 ==
  Current Measurement : powerlib/Measurements/Current Measurement  PhasorSimulation=on  OutputType=Complex  PSBequivalent=0
  Current Measurement1 : powerlib/Measurements/Current Measurement  PhasorSimulation=on  OutputType=Complex  PSBequivalent=0
  Current Measurement2 : powerlib/Measurements/Current Measurement  PhasorSimulation=on  OutputType=Complex  PSBequivalent=0
  Gain : Gain
  Gain1 : Gain
  Ground : powerlib/Elements/Ground  LConnTagsString=a
  Ground1 : powerlib/Elements/Ground  LConnTagsString=a
  Ground2 : powerlib/Elements/Ground  LConnTagsString=a
  Mux : Mux  Inputs=3
  Mux1 : Mux  Inputs=3
  Voltage Measurement : powerlib/Measurements/Voltage Measurement  PhasorSimulation=on  OutputType=Complex  PSBequivalent=0
  Voltage Measurement1 : powerlib/Measurements/Voltage Measurement  PhasorSimulation=on  OutputType=Complex  PSBequivalent=0
  Voltage Measurement2 : powerlib/Measurements/Voltage Measurement  PhasorSimulation=on  OutputType=Complex  PSBequivalent=0
  A : PMIOPort  Side=Left
  B : PMIOPort  Port=2  Side=Left
  C : PMIOPort  Port=3  Side=Left
  a : PMIOPort  Port=4  Side=Right
  b : PMIOPort  Port=5  Side=Right
  c : PMIOPort  Port=6  Side=Right
  tag scope: I10=global, V10=global
  wires:
  Voltage Measurement2/1 -> Mux/3
  Voltage Measurement1/1 -> Mux/2
  Voltage Measurement/1 -> Mux/1
  Current Measurement/1 -> Mux1/1
  Current Measurement1/1 -> Mux1/2
  Current Measurement2/1 -> Mux1/3
  Mux/1 -> Gain/1
  Gain/1 -> [V10]
  Mux1/1 -> Gain1/1
  Gain1/1 -> [I10]
  connections:
  Current Measurement/RConn1 -- a/RConn1
  Current Measurement1/LConn1 -- Voltage Measurement1/LConn1 -- B/RConn1
  Current Measurement2/LConn1 -- Voltage Measurement2/LConn1 -- C/RConn1
  A/RConn1 -- Current Measurement/LConn1 -- Voltage Measurement/LConn1
  Current Measurement1/RConn1 -- b/RConn1
  Current Measurement2/RConn1 -- c/RConn1
  Ground/LConn1 -- Voltage Measurement/LConn2
  Ground1/LConn1 -- Voltage Measurement1/LConn2
  Ground2/LConn1 -- Voltage Measurement2/LConn2

== system Scenario_3_PF/B11 ==
  Current Measurement : powerlib/Measurements/Current Measurement  PhasorSimulation=on  OutputType=Complex  PSBequivalent=0
  Current Measurement1 : powerlib/Measurements/Current Measurement  PhasorSimulation=on  OutputType=Complex  PSBequivalent=0
  Current Measurement2 : powerlib/Measurements/Current Measurement  PhasorSimulation=on  OutputType=Complex  PSBequivalent=0
  Gain : Gain
  Gain1 : Gain
  Ground : powerlib/Elements/Ground  LConnTagsString=a
  Ground1 : powerlib/Elements/Ground  LConnTagsString=a
  Ground2 : powerlib/Elements/Ground  LConnTagsString=a
  Mux : Mux  Inputs=3
  Mux1 : Mux  Inputs=3
  Voltage Measurement : powerlib/Measurements/Voltage Measurement  PhasorSimulation=on  OutputType=Complex  PSBequivalent=0
  Voltage Measurement1 : powerlib/Measurements/Voltage Measurement  PhasorSimulation=on  OutputType=Complex  PSBequivalent=0
  Voltage Measurement2 : powerlib/Measurements/Voltage Measurement  PhasorSimulation=on  OutputType=Complex  PSBequivalent=0
  A : PMIOPort  Side=Left
  B : PMIOPort  Port=2  Side=Left
  C : PMIOPort  Port=3  Side=Left
  a : PMIOPort  Port=4  Side=Right
  b : PMIOPort  Port=5  Side=Right
  c : PMIOPort  Port=6  Side=Right
  tag scope: I11=global, V11=global
  wires:
  Voltage Measurement2/1 -> Mux/3
  Voltage Measurement1/1 -> Mux/2
  Voltage Measurement/1 -> Mux/1
  Current Measurement/1 -> Mux1/1
  Current Measurement1/1 -> Mux1/2
  Current Measurement2/1 -> Mux1/3
  Mux/1 -> Gain/1
  Gain/1 -> [V11]
  Mux1/1 -> Gain1/1
  Gain1/1 -> [I11]
  connections:
  Current Measurement/RConn1 -- a/RConn1
  Current Measurement1/LConn1 -- Voltage Measurement1/LConn1 -- B/RConn1
  Current Measurement2/LConn1 -- Voltage Measurement2/LConn1 -- C/RConn1
  A/RConn1 -- Current Measurement/LConn1 -- Voltage Measurement/LConn1
  Current Measurement1/RConn1 -- b/RConn1
  Current Measurement2/RConn1 -- c/RConn1
  Ground/LConn1 -- Voltage Measurement/LConn2
  Ground1/LConn1 -- Voltage Measurement1/LConn2
  Ground2/LConn1 -- Voltage Measurement2/LConn2

== system Scenario_3_PF/B12 ==
  Current Measurement : powerlib/Measurements/Current Measurement  PhasorSimulation=on  OutputType=Complex  PSBequivalent=0
  Current Measurement1 : powerlib/Measurements/Current Measurement  PhasorSimulation=on  OutputType=Complex  PSBequivalent=0
  Current Measurement2 : powerlib/Measurements/Current Measurement  PhasorSimulation=on  OutputType=Complex  PSBequivalent=0
  Gain : Gain
  Gain1 : Gain
  Ground : powerlib/Elements/Ground  LConnTagsString=a
  Ground1 : powerlib/Elements/Ground  LConnTagsString=a
  Ground2 : powerlib/Elements/Ground  LConnTagsString=a
  Mux : Mux  Inputs=3
  Mux1 : Mux  Inputs=3
  Voltage Measurement : powerlib/Measurements/Voltage Measurement  PhasorSimulation=on  OutputType=Complex  PSBequivalent=0
  Voltage Measurement1 : powerlib/Measurements/Voltage Measurement  PhasorSimulation=on  OutputType=Complex  PSBequivalent=0
  Voltage Measurement2 : powerlib/Measurements/Voltage Measurement  PhasorSimulation=on  OutputType=Complex  PSBequivalent=0
  A : PMIOPort  Side=Left
  B : PMIOPort  Port=2  Side=Left
  C : PMIOPort  Port=3  Side=Left
  a : PMIOPort  Port=4  Side=Right
  b : PMIOPort  Port=5  Side=Right
  c : PMIOPort  Port=6  Side=Right
  tag scope: I12=global, V12=global
  wires:
  Voltage Measurement2/1 -> Mux/3
  Voltage Measurement1/1 -> Mux/2
  Voltage Measurement/1 -> Mux/1
  Current Measurement/1 -> Mux1/1
  Current Measurement1/1 -> Mux1/2
  Current Measurement2/1 -> Mux1/3
  Mux/1 -> Gain/1
  Gain/1 -> [V12]
  Mux1/1 -> Gain1/1
  Gain1/1 -> [I12]
  connections:
  Current Measurement/RConn1 -- a/RConn1
  Current Measurement1/LConn1 -- Voltage Measurement1/LConn1 -- B/RConn1
  Current Measurement2/LConn1 -- Voltage Measurement2/LConn1 -- C/RConn1
  A/RConn1 -- Current Measurement/LConn1 -- Voltage Measurement/LConn1
  Current Measurement1/RConn1 -- b/RConn1
  Current Measurement2/RConn1 -- c/RConn1
  Ground/LConn1 -- Voltage Measurement/LConn2
  Ground1/LConn1 -- Voltage Measurement1/LConn2
  Ground2/LConn1 -- Voltage Measurement2/LConn2

== system Scenario_3_PF/B13 ==
  Current Measurement : powerlib/Measurements/Current Measurement  PhasorSimulation=on  OutputType=Complex  PSBequivalent=0
  Current Measurement1 : powerlib/Measurements/Current Measurement  PhasorSimulation=on  OutputType=Complex  PSBequivalent=0
  Current Measurement2 : powerlib/Measurements/Current Measurement  PhasorSimulation=on  OutputType=Complex  PSBequivalent=0
  Gain : Gain
  Gain1 : Gain
  Ground : powerlib/Elements/Ground  LConnTagsString=a
  Ground1 : powerlib/Elements/Ground  LConnTagsString=a
  Ground2 : powerlib/Elements/Ground  LConnTagsString=a
  Mux : Mux  Inputs=3
  Mux1 : Mux  Inputs=3
  Voltage Measurement : powerlib/Measurements/Voltage Measurement  PhasorSimulation=on  OutputType=Complex  PSBequivalent=0
  Voltage Measurement1 : powerlib/Measurements/Voltage Measurement  PhasorSimulation=on  OutputType=Complex  PSBequivalent=0
  Voltage Measurement2 : powerlib/Measurements/Voltage Measurement  PhasorSimulation=on  OutputType=Complex  PSBequivalent=0
  A : PMIOPort  Side=Left
  B : PMIOPort  Port=2  Side=Left
  C : PMIOPort  Port=3  Side=Left
  a : PMIOPort  Port=4  Side=Right
  b : PMIOPort  Port=5  Side=Right
  c : PMIOPort  Port=6  Side=Right
  tag scope: I13=global, V13=global
  wires:
  Voltage Measurement2/1 -> Mux/3
  Voltage Measurement1/1 -> Mux/2
  Voltage Measurement/1 -> Mux/1
  Current Measurement/1 -> Mux1/1
  Current Measurement1/1 -> Mux1/2
  Current Measurement2/1 -> Mux1/3
  Mux/1 -> Gain/1
  Gain/1 -> [V13]
  Mux1/1 -> Gain1/1
  Gain1/1 -> [I13]
  connections:
  Current Measurement/RConn1 -- a/RConn1
  Current Measurement1/LConn1 -- Voltage Measurement1/LConn1 -- B/RConn1
  Current Measurement2/LConn1 -- Voltage Measurement2/LConn1 -- C/RConn1
  A/RConn1 -- Current Measurement/LConn1 -- Voltage Measurement/LConn1
  Current Measurement1/RConn1 -- b/RConn1
  Current Measurement2/RConn1 -- c/RConn1
  Ground/LConn1 -- Voltage Measurement/LConn2
  Ground1/LConn1 -- Voltage Measurement1/LConn2
  Ground2/LConn1 -- Voltage Measurement2/LConn2
